simulink model "WindFoR_model"  (R2024a)
settings: Solver=VariableStepAuto  StartTime=0.0  StopTime=10.0  RelTol=1e-3
values from neighbouring files (symbols this model uses):
  b = 37.4*0.3048    (= 11.39952)    [a1_initialize.m]
  cbar = 11.52*0.3048    (= 3.511296)    [a1_initialize.m]
  g = 9.80665    [a1_initialize.m]
  InertiaTensor = [Ixx 0 -Ixz; 0 Iyy 0; -Ixz 0 Izz]    [a1_initialize.m]
  init_eulers = x0(7:9)    [a1_initialize.m]
  init_inertial = x0(10:12)    [a1_initialize.m]
  mass = 36100/2.2046    (= 16374.852581)    [a1_initialize.m]
  max_thrust = 32000*g/2.2046    (= 142344.5523)    [a1_initialize.m]
  S = 400.0*0.3048*0.3048    (= 37.161216)    [a1_initialize.m]
undefined symbols (not defined in the file or in its folder): CD0, CDalpha, CDelevator, CL0, Clalieron, CLalpha, CLalpha_dot, Clbeta, CLelevator, Clp, CLq, Clr, Clrudder, Cm0, Cmalpha, Cmalpha_dot, Cmelevator, Cmq, Cnalieron, Cnbeta, Cnp, Cnr, Cnrudder, CYalieron, CYbeta, CYp, CYr, CYrudder
libraries: Rotation_Matrices_All x2, matrix_library x2
settings Model: Creator=ragup  LastModifiedBy=ragup

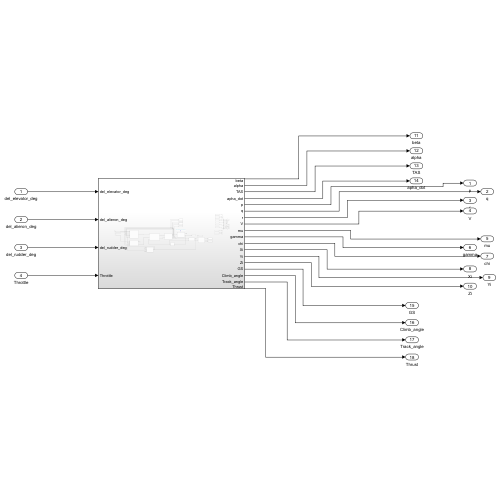
[thumbnail: Simulink's stored preview of the top-level diagram]
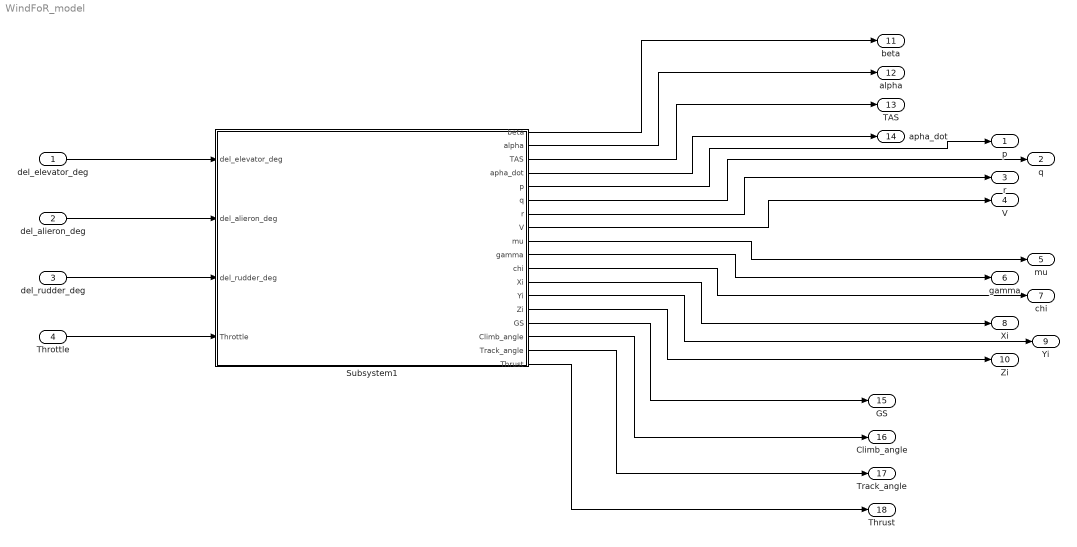
== system WindFoR_model ==
  del_elevator_deg : Inport
  del_alieron_deg : Inport  Port=2
  del_rudder_deg : Inport  Port=3
  Throttle : Inport  Port=4
  Subsystem1 : Subsystem
  p : Outport
  q : Outport  Port=2
  r : Outport  Port=3
  V : Outport  Port=4
  mu : Outport  Port=5
  gamma : Outport  Port=6
  chi : Outport  Port=7
  Xi : Outport  Port=8
  Yi : Outport  Port=9
  Zi : Outport  Port=10
  beta : Outport  Port=11
  alpha : Outport  Port=12
  TAS : Outport  Port=13
  apha_dot : Outport  Port=14
  GS : Outport  Port=15
  Climb_angle : Outport  Port=16
  Track_angle : Outport  Port=17
  Thrust : Outport  Port=18
  wires:
  del_elevator_deg/1 -> Subsystem1/1(del_elevator_deg)
  del_alieron_deg/1 -> Subsystem1/2(del_alieron_deg)
  del_rudder_deg/1 -> Subsystem1/3(del_rudder_deg)
  Throttle/1 -> Subsystem1/4(Throttle)
  Subsystem1/1(beta) -> beta/1
  Subsystem1/2(alpha) -> alpha/1
  Subsystem1/3(TAS) -> TAS/1
  Subsystem1/4(apha_dot) -> apha_dot/1
  Subsystem1/5(p) -> p/1
  Subsystem1/6(q) -> q/1
  Subsystem1/7(r) -> r/1
  Subsystem1/8(V) -> V/1
  Subsystem1/9(mu) -> mu/1
  Subsystem1/10(gamma) -> gamma/1
  Subsystem1/11(chi) -> chi/1
  Subsystem1/12(Xi) -> Xi/1
  Subsystem1/13(Yi) -> Yi/1
  Subsystem1/14(Zi) -> Zi/1
  Subsystem1/15(GS) -> GS/1
  Subsystem1/16(Climb_angle) -> Climb_angle/1
  Subsystem1/17(Track_angle) -> Track_angle/1
  Subsystem1/18(Thrust) -> Thrust/1

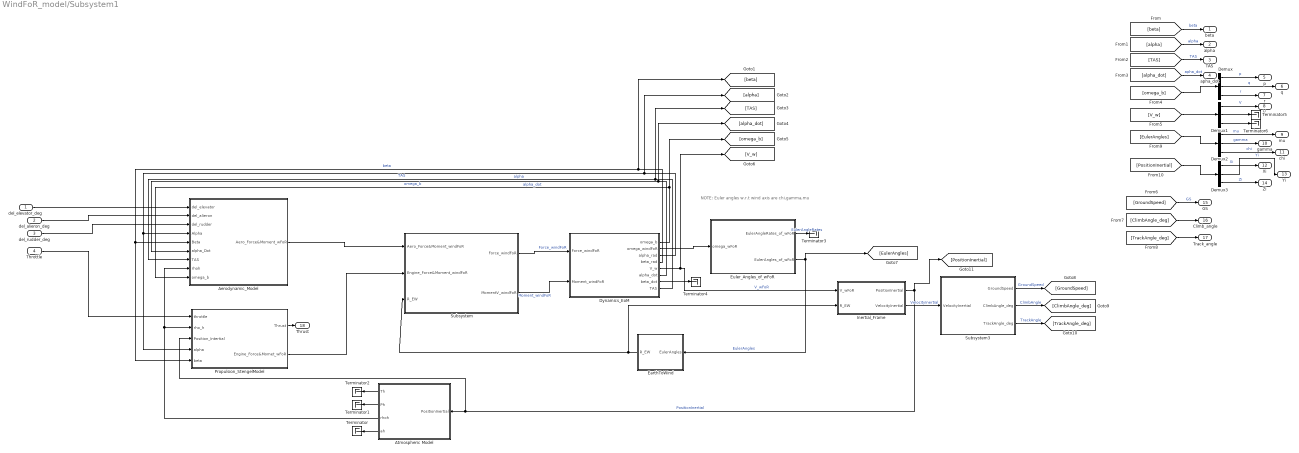
== system WindFoR_model/Subsystem1 ==
  note: NOTE: Euler angles w.r.t wind axis are chi,gamma,mu
  del_elevator_deg : Inport
  del_alieron_deg : Inport  Port=2
  del_rudder_deg : Inport  Port=3
  Throttle : Inport  Port=4
  Aerodynamic_Model : Subsystem
  Atmospheric Model : Subsystem
  Demux{,1..3} (4 alike) : Demux  Outputs=3
  Dynamics_EoM : Subsystem
  EarthToWind : Subsystem
  Euler_Angles_of_wFoR : Subsystem
  Inertial_Frame : Subsystem
  Propulsion_StengelModel : Subsystem
  Subsystem : Subsystem
  Subsystem3 : Subsystem
  Terminator{,1..6} (7 alike) : Terminator
  beta : Outport
  alpha : Outport  Port=2
  TAS : Outport  Port=3
  apha_dot : Outport  Port=4
  p : Outport  Port=5
  q : Outport  Port=6
  r : Outport  Port=7
  V : Outport  Port=8
  mu : Outport  Port=9
  gamma : Outport  Port=10
  chi : Outport  Port=11
  Xi : Outport  Port=12
  Yi : Outport  Port=13
  Zi : Outport  Port=14
  GS : Outport  Port=15
  Climb_angle : Outport  Port=16
  Track_angle : Outport  Port=17
  Thrust : Outport  Port=18
  wires:
  [alpha] -> alpha/1  "alpha"
  [EulerAngles] -> Demux2/1
  Dynamics_EoM/5(V_w) -> [V_w], Inertial_Frame/1(V_wFoR)  "V_wFoR"
  Dynamics_EoM/8(TAS) -> [TAS], Aerodynamic_Model/7(TAS)  "TAS"
  Euler_Angles_of_wFoR/2(EulerAngles_of_wFoR) -> [EulerAngles], EarthToWind/1(EulerAngles)  "EulerAngles"
  [beta] -> beta/1  "beta"
  Dynamics_EoM/4(beta_rad) -> [beta], Aerodynamic_Model/5(Beta), Propulsion_StengelModel/5(beta)  "beta"
  Propulsion_StengelModel/1(Thrust) -> Thrust/1
  Dynamics_EoM/3(alpha_rad) -> [alpha], Aerodynamic_Model/4(Alpha), Propulsion_StengelModel/4(alpha)  "alpha"
  Atmospheric Model/2(Ph) -> Terminator1/1
  Demux1/2 -> Terminator5/1
  Atmospheric Model/4(ah) -> Terminator/1
  [TrackAngle_deg] -> Track_angle/1
  [GroundSpeed] -> GS/1  "GS"
  Dynamics_EoM/7(beta_dot) -> Terminator4/1
  Subsystem3/2(ClimbAngle_deg) -> [ClimbAngle_deg]  "ClimbAngle"
  Demux/3 -> r/1  "r"
  [omega_b] -> Demux/1
  Atmospheric Model/1(Th) -> Terminator2/1
  Demux1/3 -> Terminator6/1
  [alpha_dot] -> apha_dot/1  "apha_dot"
  Demux3/2 -> Yi/1  "Yi"
  Subsystem/1(Force_windFoR) -> Dynamics_EoM/1(Force_windFoR)  "Force_windFoR"
  Demux2/2 -> gamma/1  "gamma"
  Demux1/1 -> V/1  "V"
  Demux/2 -> q/1  "q"
  [PositionInertial] -> Demux3/1
  Demux3/1 -> Xi/1  "Xi"
  del_alieron_deg/1 -> Aerodynamic_Model/2(del_alieron)
  Atmospheric Model/3(rhoh) -> Propulsion_StengelModel/2(rho_h), Aerodynamic_Model/8(rhoh)
  Euler_Angles_of_wFoR/1(EulerAngleRates_of_wFoR) -> Terminator3/1  "EulerAngleRates"
  Subsystem3/1(GroundSpeed) -> [GroundSpeed]  "GroundSpeed"
  Demux2/3 -> chi/1  "chi"
  Dynamics_EoM/1(omega_b) -> [omega_b], Aerodynamic_Model/9(omega_b)  "omega_b"
  Propulsion_StengelModel/2(Engine_Force&Momet_wFoR) -> Subsystem/2(Engine_Force&Moment_windFoR)
  Demux2/1 -> mu/1  "mu"
  Dynamics_EoM/6(alpha_dot) -> [alpha_dot], Aerodynamic_Model/6(alpha_Dot)  "alpha_dot"
  del_elevator_deg/1 -> Aerodynamic_Model/1(del_elevator)
  Inertial_Frame/2(VelocityInertial) -> Subsystem3/1(VelocityInertial)  "VelocityInertial"
  del_rudder_deg/1 -> Aerodynamic_Model/3(del_rudder)
  EarthToWind/1(R_EW) -> Inertial_Frame/2(R_EW), Subsystem/3(R_EW)
  Subsystem/2(MomentV_windFoR) -> Dynamics_EoM/2(Moment_windFoR)  "Moment_windFoR"
  Demux3/3 -> Zi/1  "Zi"
  Aerodynamic_Model/1(Aero_Force&Moment_wFoR) -> Subsystem/1(Aero_Force&Moment_windFoR)
  [TAS] -> TAS/1  "TAS"
  Subsystem3/3(TrackAngle_deg) -> [TrackAngle_deg]  "TrackAngle"
  Inertial_Frame/1(PositionInertial) -> [PositionInertial], Propulsion_StengelModel/3(Position_Intertial), Atmospheric Model/1(PositionInertial)  "PositionInertial"
  Dynamics_EoM/2(omega_windFoR) -> Euler_Angles_of_wFoR/1(omega_wFoR)
  [ClimbAngle_deg] -> Climb_angle/1
  Throttle/1 -> Propulsion_StengelModel/1(throttle)
  [V_w] -> Demux1/1
  Demux/1 -> p/1  "p"

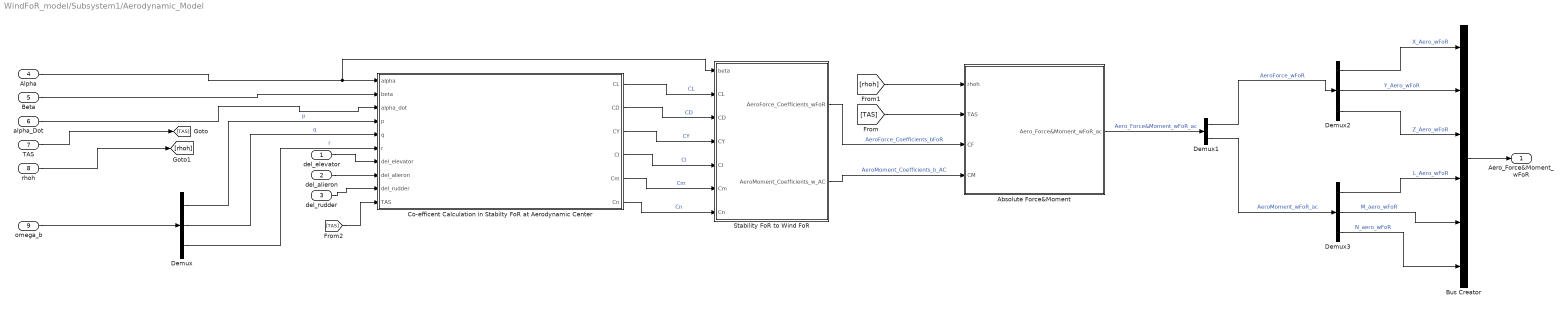
== system WindFoR_model/Subsystem1/Aerodynamic_Model ==
  del_elevator : Inport
  del_alieron : Inport  Port=2
  del_rudder : Inport  Port=3
  Alpha : Inport  Port=4
  Beta : Inport  Port=5
  alpha_Dot : Inport  Port=6
  TAS : Inport  Port=7
  rhoh : Inport  Port=8
  omega_b : Inport  Port=9
  Absolute Force&Moment : Subsystem
  Bus Creator : BusCreator  Inputs=6
  Co-efficent Calculation in Stabilty FoR at Aerodynamic Center : Subsystem
  Demux : Demux  Outputs=3
  Demux1 : Demux  Outputs=2
  Demux2 : Demux  Outputs=3
  Demux3 : Demux  Outputs=3
  Stability FoR to Wind FoR : Subsystem
  Aero_Force&Moment_wFoR : Outport
  wires:
  Demux/1 -> Co-efficent Calculation in Stabilty FoR at Aerodynamic Center/4(p)  "p"
  omega_b/1 -> Demux/1
  [TAS] -> Co-efficent Calculation in Stabilty FoR at Aerodynamic Center/10(TAS)
  TAS/1 -> [TAS]
  rhoh/1 -> [rhoh]
  Demux/2 -> Co-efficent Calculation in Stabilty FoR at Aerodynamic Center/5(q)  "q"
  Alpha/1 -> Stability FoR to Wind FoR/1(beta), Co-efficent Calculation in Stabilty FoR at Aerodynamic Center/1(alpha)
  Co-efficent Calculation in Stabilty FoR at Aerodynamic Center/1(CL) -> Stability FoR to Wind FoR/2(CL)  "CL"
  Co-efficent Calculation in Stabilty FoR at Aerodynamic Center/6(Cn) -> Stability FoR to Wind FoR/7(Cn)  "Cn"
  del_alieron/1 -> Co-efficent Calculation in Stabilty FoR at Aerodynamic Center/8(del_alieron)
  alpha_Dot/1 -> Co-efficent Calculation in Stabilty FoR at Aerodynamic Center/3(alpha_dot)
  Co-efficent Calculation in Stabilty FoR at Aerodynamic Center/3(CY) -> Stability FoR to Wind FoR/4(CY)  "CY"
  Co-efficent Calculation in Stabilty FoR at Aerodynamic Center/5(Cm) -> Stability FoR to Wind FoR/6(Cm)  "Cm"
  Co-efficent Calculation in Stabilty FoR at Aerodynamic Center/2(CD) -> Stability FoR to Wind FoR/3(CD)  "CD"
  Co-efficent Calculation in Stabilty FoR at Aerodynamic Center/4(Cl) -> Stability FoR to Wind FoR/5(Cl)  "Cl"
  Stability FoR to Wind FoR/1(AeroForce_Coefficients_wFoR) -> Absolute Force&Moment/3(CF)  "AeroForce_Coefficients_bFoR"
  [TAS] -> Absolute Force&Moment/2(TAS)
  [rhoh] -> Absolute Force&Moment/1(rhoh)
  Demux/3 -> Co-efficent Calculation in Stabilty FoR at Aerodynamic Center/6(r)  "r"
  del_elevator/1 -> Co-efficent Calculation in Stabilty FoR at Aerodynamic Center/7(del_elevator)
  Beta/1 -> Co-efficent Calculation in Stabilty FoR at Aerodynamic Center/2(beta)
  del_rudder/1 -> Co-efficent Calculation in Stabilty FoR at Aerodynamic Center/9(del_rudder)
  Stability FoR to Wind FoR/2(AeroMoment_Coefficients_w_AC) -> Absolute Force&Moment/4(CM)  "AeroMoment_Coefficients_b_AC"
  Absolute Force&Moment/1(Aero_Force&Moment_wFoR_ac) -> Demux1/1  "Aero_Force&Moment_wFoR_ac"
  Demux1/1 -> Demux2/1  "AeroForce_wFoR"
  Demux1/2 -> Demux3/1  "AeroMoment_wFoR_ac"
  Demux2/1 -> Bus Creator/1  "X_Aero_wFoR"
  Demux2/2 -> Bus Creator/2  "Y_Aero_wFoR"
  Demux2/3 -> Bus Creator/3  "Z_Aero_wFoR"
  Demux3/2 -> Bus Creator/5  "M_aero_wFoR"
  Demux3/1 -> Bus Creator/4  "L_Aero_wFoR"
  Demux3/3 -> Bus Creator/6  "N_aero_wFoR"
  Bus Creator/1 -> Aero_Force&Moment_wFoR/1

== system WindFoR_model/Subsystem1/Atmospheric Model ==
  PositionInertial : Inport
  Demux : Demux  Outputs=3
  Gain : Gain  Gain=-1
  ISA_upto20km : Subsystem
      mask Display: image('ISA_Temperature.png', [3,3,3,3,100,100]);
  Terminator : Terminator
  Terminator1 : Terminator
  Th : Outport
  Ph : Outport  Port=2
  rhoh : Outport  Port=3
  ah : Outport  Port=4
  wires:
  Demux/3 -> Gain/1
  PositionInertial/1 -> Demux/1
  ISA_upto20km/3(rhoh) -> rhoh/1  "rhoh"
  Gain/1 -> ISA_upto20km/1(h)
  Demux/2 -> Terminator1/1
  Demux/1 -> Terminator/1
  ISA_upto20km/1(Th) -> Th/1  "Th"
  ISA_upto20km/2(Ph) -> Ph/1  "Ph"
  ISA_upto20km/4(ah) -> ah/1  "ah"

== system WindFoR_model/Subsystem1/Dynamics_EoM ==
  Force_windFoR : Inport
  Moment_windFoR : Inport  Port=2
  Force_Dynamics_WindAxis : Subsystem
  Moment_Dynamics_bodyFoR : Subsystem
  Product1 : Product  Multiplication=Matrix(*)
  omega_b : Outport
  omega_windFoR : Outport  Port=2
  alpha_rad : Outport  Port=3
  beta_rad : Outport  Port=4
  V_w : Outport  Port=5
  alpha_dot : Outport  Port=6
  beta_dot : Outport  Port=7
  TAS : Outport  Port=8
  wires:
  Force_Dynamics_WindAxis/1(omega_w) -> omega_windFoR/1
  Moment_Dynamics_bodyFoR/1(omega_b) -> omega_b/1, Force_Dynamics_WindAxis/1(omega_b)  "omega_b"
  Force_Dynamics_WindAxis/8(beta_dot) -> beta_dot/1
  Force_Dynamics_WindAxis/7(alpha_dot) -> alpha_dot/1
  Force_Dynamics_WindAxis/5(V_w) -> V_w/1
  Force_Dynamics_WindAxis/4(beta_rad) -> beta_rad/1
  Force_Dynamics_WindAxis/3(alpha_rad) -> alpha_rad/1
  Product1/1 -> Moment_Dynamics_bodyFoR/1(Moment_bodyFoR)  "Moment_bodyFoR"
  Force_Dynamics_WindAxis/2(R_wb) -> [R_wb]
  Force_windFoR/1 -> Force_Dynamics_WindAxis/2(Force_w)  "Force_windFoR"
  [R_wb] -> Product1/1  "R_WB"
  Moment_windFoR/1 -> Product1/2
  Force_Dynamics_WindAxis/6(TAS) -> TAS/1

== system WindFoR_model/Subsystem1/EarthToWind ==
  EulerAngles : Inport
  Demux : Demux  Outputs=3
  Product1 : Product  Multiplication=Matrix(*)
  Product2 : Product  Multiplication=Matrix(*)
  Subsystem2 : Subsystem
  Subsystem3 : Subsystem
  Subsystem4 : Subsystem
  R_EW : Outport
  wires:
  Demux/3 -> Subsystem2/1(chi)  "chi"
  Demux/2 -> Subsystem4/1(gamma)  "gamma"
  EulerAngles/1 -> Demux/1  "EulerAngles"
  Demux/1 -> Subsystem3/1(mu)  "mu"
  Product2/1 -> R_EW/1
  Product1/1 -> Product2/1
  Subsystem2/1(R_chi) -> Product2/2
  Subsystem4/1(R_gamma) -> Product1/2
  Subsystem3/1(R_mu) -> Product1/1

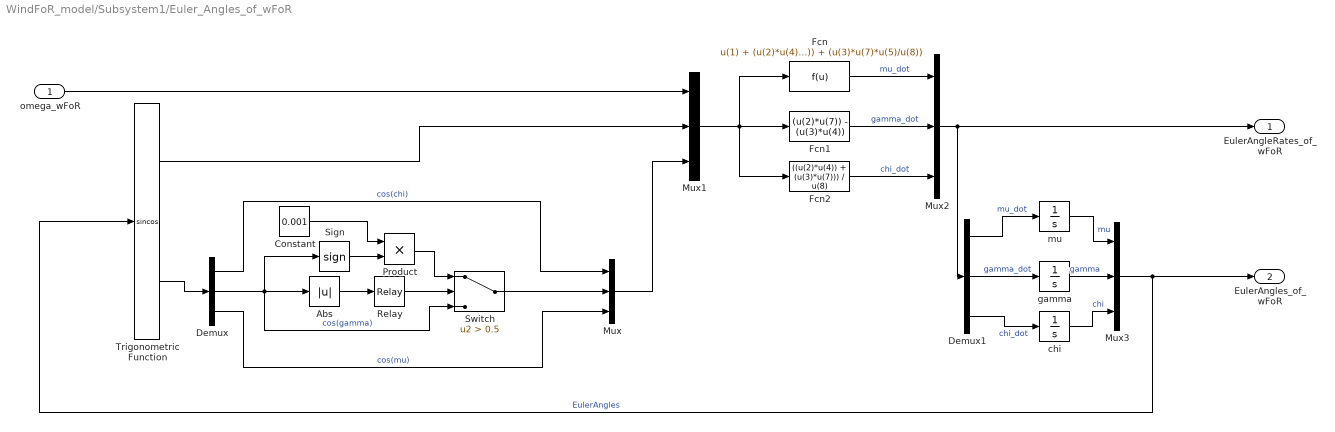
== system WindFoR_model/Subsystem1/Euler_Angles_of_wFoR ==
  omega_wFoR : Inport
  Abs : Abs  SaturateOnIntegerOverflow=off
  Constant : Constant  Value=0.001
  Demux : Demux  Outputs=3
  Demux1 : Demux  Outputs=3
  Fcn : Fcn  Expr=u(1) + (u(2)*u(4)*u(5)/u(8)) + (u(3)*u(7)*u(5)/u(8))
  Fcn1 : Fcn  Expr=(u(2)*u(7)) - (u(3)*u(4))
  Fcn2 : Fcn  Expr=((u(2)*u(4)) + (u(3)*u(7))) / u(8)
  Mux{,1..3} (4 alike) : Mux  Inputs=3
  Product : Product
  Relay : Relay  OnSwitchValue=0.001  OffSwitchValue=0  OnOutputValue=0  OffOutputValue=1
  Sign : Signum
  Switch : Switch  Criteria=u2 > Threshold  Threshold=0.5  SaturateOnIntegerOverflow=off  InputSameDT=off
  Trigonometric Function : Trigonometry  Operator=sincos
  chi : Integrator  InitialCondition=init_eulers(3)  ContinuousStateAttributes='chi'
  gamma : Integrator  InitialCondition=init_eulers(2)  ContinuousStateAttributes='gamma'
  mu : Integrator  InitialCondition=init_eulers(1)  ContinuousStateAttributes='mu'
  EulerAngleRates_of_wFoR : Outport
  EulerAngles_of_wFoR : Outport  Port=2
  wires:
  Mux3/1 -> EulerAngles_of_wFoR/1, Trigonometric Function/1  "EulerAngles"
  mu/1 -> Mux3/1  "mu"
  Demux1/3 -> chi/1  "chi_dot"
  Mux2/1 -> Demux1/1, EulerAngleRates_of_wFoR/1
  Demux1/2 -> gamma/1  "gamma_dot"
  gamma/1 -> Mux3/2  "gamma"
  Demux1/1 -> mu/1  "mu_dot"
  chi/1 -> Mux3/3  "chi"
  Fcn2/1 -> Mux2/3  "chi_dot"
  Mux/1 -> Mux1/3
  Constant/1 -> Product/1
  Demux/1 -> Mux/1  "cos(chi)"
  Fcn1/1 -> Mux2/2  "gamma_dot"
  Demux/3 -> Mux/3  "cos(mu)"
  Switch/1 -> Mux/2
  Mux1/1 -> Fcn1/1, Fcn2/1, Fcn/1
  Sign/1 -> Product/2
  Abs/1 -> Relay/1
  Fcn/1 -> Mux2/1  "mu_dot"
  Relay/1 -> Switch/2
  Product/1 -> Switch/1
  omega_wFoR/1 -> Mux1/1
  Trigonometric Function/2 -> Demux/1
  Trigonometric Function/1 -> Mux1/2
  Demux/2 -> Abs/1, Switch/3, Sign/1  "cos(gamma)"

== system WindFoR_model/Subsystem1/Inertial_Frame ==
  V_wFoR : Inport
  R_EW : Inport  Port=2
  Demux : Demux  Outputs=3
  Matrix Multiply : Product  Multiplication=Matrix(*)
  Mux : Mux  Inputs=3
  Transpose : Math  Operator=transpose
  Xi_dot : Integrator  InitialCondition=init_inertial(1)  ContinuousStateAttributes='Xi_dot'
  Yi_dot : Integrator  InitialCondition=init_inertial(2)  ContinuousStateAttributes='Yi_dot'
  Zi_dot : Integrator  InitialCondition=init_inertial(3)  ContinuousStateAttributes='Zi_dot'
  PositionInertial : Outport
  VelocityInertial : Outport  Port=2
  wires:
  R_EW/1 -> Transpose/1
  Matrix Multiply/1 -> Demux/1, VelocityInertial/1
  Transpose/1 -> Matrix Multiply/1  "R_WE"
  V_wFoR/1 -> Matrix Multiply/2
  Demux/3 -> Zi_dot/1  "Zi_dot"
  Mux/1 -> PositionInertial/1
  Zi_dot/1 -> Mux/3  "Zi"
  Xi_dot/1 -> Mux/1  "Xi"
  Demux/1 -> Xi_dot/1  "Xi_dot"
  Demux/2 -> Yi_dot/1  "Yi_dot"
  Yi_dot/1 -> Mux/2  "Yi"

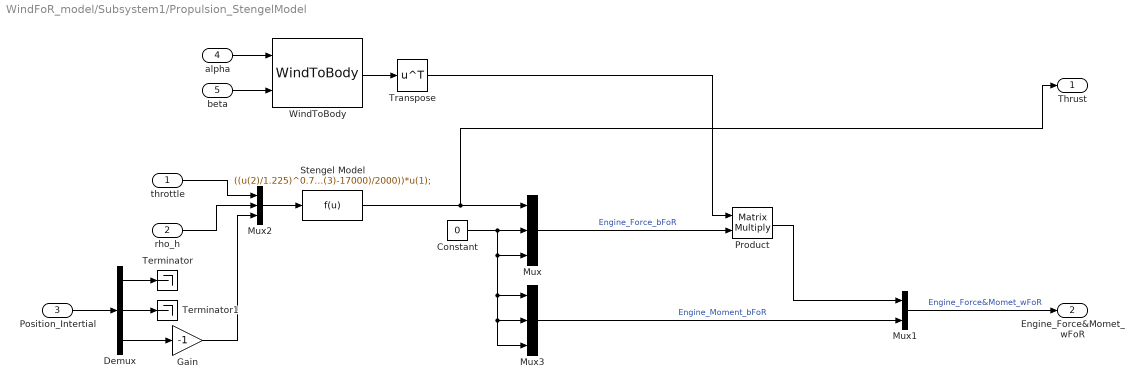
== system WindFoR_model/Subsystem1/Propulsion_StengelModel ==
  throttle : Inport
  rho_h : Inport  Port=2
  Position_Intertial : Inport  Port=3
  alpha : Inport  Port=4
  beta : Inport  Port=5
  Constant : Constant  Value=0
  Demux : Demux  Outputs=3
  Gain : Gain  Gain=-1
  Mux : Mux  Inputs=3
  Mux1 : Mux  Inputs=2
  Mux2 : Mux  Inputs=3
  Mux3 : Mux  Inputs=3
  Product : Product  Multiplication=Matrix(*)
  Stengel Model : Fcn  Expr=((u(2)/1.225)^0.7)*max_thrust*(1-exp((u(3)-17000)/2000))*u(1);
  Terminator : Terminator
  Terminator1 : Terminator
  Transpose : Math  Operator=transpose
  WindToBody : Rotation_Matrices_All/WindToBody  SystemSampleTime=-1  VariantActivationTime=update diagram  AllowFlexibleInterface=on  Latency=0  AutoFrameSizeCalculation=off
  Thrust : Outport
  Engine_Force&Momet_wFoR : Outport  Port=2
  wires:
  Stengel Model/1 -> Thrust/1, Mux/1
  Constant/1 -> Mux3/3, Mux3/2, Mux3/1, Mux/3, Mux/2
  Mux/1 -> Product/2  "Engine_Force_bFoR"
  Mux2/1 -> Stengel Model/1
  throttle/1 -> Mux2/1
  rho_h/1 -> Mux2/2
  Gain/1 -> Mux2/3
  Demux/3 -> Gain/1
  Demux/1 -> Terminator/1
  Demux/2 -> Terminator1/1
  Position_Intertial/1 -> Demux/1
  WindToBody/1 -> Transpose/1
  Transpose/1 -> Product/1
  Product/1 -> Mux1/1
  Mux1/1 -> Engine_Force&Momet_wFoR/1  "Engine_Force&Momet_wFoR"
  Mux3/1 -> Mux1/2  "Engine_Moment_bFoR"
  alpha/1 -> WindToBody/1
  beta/1 -> WindToBody/2

== system WindFoR_model/Subsystem1/Subsystem ==
  Aero_Force&Moment_windFoR : Inport
  Engine_Force&Moment_windFoR : Inport  Port=2
  R_EW : Inport  Port=3
  Add : Sum
  Constant : Constant  Value=0
  Constant1 : Constant  Value=mass
  Demux : Demux  Outputs=2
  Gain : Gain  Gain=g
  Mux : Mux  Inputs=3
  Product : Product  Multiplication=Matrix(*)
  Sum : Sum  Inputs=|++
  Force_windFoR : Outport
  MomentV_windFoR : Outport  Port=2
  wires:
  Mux/1 -> Product/2
  Demux/2 -> MomentV_windFoR/1  "Moment_windFoR"
  Add/1 -> Demux/1
  Product/1 -> Sum/1  "Gravity_Force_windFoR"
  Engine_Force&Moment_windFoR/1 -> Add/2
  Sum/1 -> Force_windFoR/1  "Force_windFoR"
  Demux/1 -> Sum/2
  Gain/1 -> Mux/3  "weight"
  Aero_Force&Moment_windFoR/1 -> Add/1
  Constant1/1 -> Gain/1
  Constant/1 -> Mux/1, Mux/2
  R_EW/1 -> Product/1

== system WindFoR_model/Subsystem1/Subsystem3 ==
  VelocityInertial : Inport
  Add : Sum
  Atan1 : Trigonometry  Operator=atan2
  Atan2 : Trigonometry  Operator=atan2
  Demux : Demux  Outputs=3
  Gain : Gain  Gain=-1
  Gain1 : Gain  Gain=180/pi
  Gain2 : Gain  Gain=180/pi
  Sqrt : Sqrt
  Square : Math  Operator=square
  Square1 : Math  Operator=square
  GroundSpeed : Outport
  ClimbAngle_deg : Outport  Port=2
  TrackAngle_deg : Outport  Port=3
  wires:
  VelocityInertial/1 -> Demux/1
  Gain/1 -> Atan2/1
  Atan1/1 -> Gain2/1
  Square/1 -> Add/1
  Demux/3 -> Gain/1  "Zdot_E"
  Add/1 -> Sqrt/1
  Atan2/1 -> Gain1/1
  Square1/1 -> Add/2
  Sqrt/1 -> Atan2/2, GroundSpeed/1
  Demux/1 -> Square/1, Atan1/2  "Xdot_E"
  Demux/2 -> Square1/1, Atan1/1  "Ydot_E"
  Gain1/1 -> ClimbAngle_deg/1
  Gain2/1 -> TrackAngle_deg/1

== system WindFoR_model/Subsystem1/Aerodynamic_Model/Absolute Force&Moment ==
  rhoh : Inport
  TAS : Inport  Port=2
  CF : Inport  Port=3
  CM : Inport  Port=4
  Constant : Constant  Value=b
  Constant1 : Constant  Value=cbar
  Demux1 : Demux  Outputs=3
  Demux2 : Demux  Outputs=3
  Mux : Mux  Inputs=6
  Product : Product
  Product1 : Product  Inputs=3
  Product2 : Product  Inputs=3
  Product3 : Product  Inputs=3
  Subsystem1 : Subsystem
  Aero_Force&Moment_wFoR_ac : Outport
  wires:
  Demux2/3 -> Product3/2
  Demux1/3 -> Mux/3  "Z_aero"
  Constant1/1 -> Product2/3
  CF/1 -> Product/2
  CM/1 -> Demux2/1
  Demux1/1 -> Mux/1  "X_aero"
  Product3/1 -> Mux/6  "N_aero"
  Subsystem1/1(QS) -> [QS]  "QS"
  Constant/1 -> Product3/3, Product1/3
  Product/1 -> Demux1/1  "Aero_Forces"
  Demux2/1 -> Product1/2  "Cl"
  Demux2/2 -> Product2/2
  [QS] -> Product3/1, Product2/1, Product1/1
  Product2/1 -> Mux/5  "M_aero"
  Demux1/2 -> Mux/2  "Y_aero"
  Product1/1 -> Mux/4  "L_aero"
  rhoh/1 -> Subsystem1/1(rhoh)
  [QS] -> Product/1
  TAS/1 -> Subsystem1/2(TAS)
  Mux/1 -> Aero_Force&Moment_wFoR_ac/1  "Aero_Force&Moment_wFoR_ac"

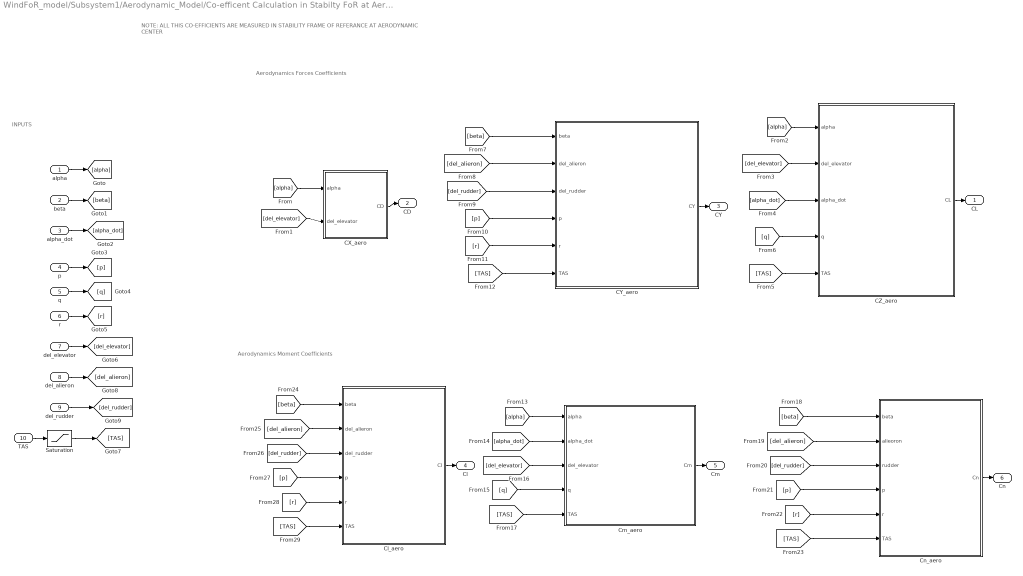
== system WindFoR_model/Subsystem1/Aerodynamic_Model/Co-efficent Calculation in Stabilty FoR at Aerodynamic Center ==
  note: INPUTS
  note: Aerodynamics Moment Coefficients
  note: Aerodynamics Forces Coefficients
  note: NOTE: ALL THIS CO-EFFICIENTS ARE MEASURED IN STABILITY FRAME OF REFERANCE AT AERODYNAMIC CENTER
  alpha : Inport
  beta : Inport  Port=2
  alpha_dot : Inport  Port=3
  p : Inport  Port=4
  q : Inport  Port=5
  r : Inport  Port=6
  del_elevator : Inport  Port=7
  del_alieron : Inport  Port=8
  del_rudder : Inport  Port=9
  TAS : Inport  Port=10
  CX_aero : Subsystem
  CY_aero : Subsystem
  CZ_aero : Subsystem
  Cl_aero : Subsystem
  Cm_aero : Subsystem
  Cn_aero : Subsystem
  Saturation : Saturate  UpperLimit=inf  LowerLimit=0.1
  CL : Outport
  CD : Outport  Port=2
  CY : Outport  Port=3
  Cl : Outport  Port=4
  Cm : Outport  Port=5
  Cn : Outport  Port=6
  wires:
  Saturation/1 -> [TAS]
  [del_elevator] -> CZ_aero/2(del_elevator)
  alpha/1 -> [alpha]
  TAS/1 -> Saturation/1
  [r] -> Cn_aero/5(r)
  [alpha] -> Cm_aero/1(alpha)
  q/1 -> [q]
  beta/1 -> [beta]
  [r] -> Cl_aero/5(r)
  del_alieron/1 -> [del_alieron]
  p/1 -> [p]
  alpha_dot/1 -> [alpha_dot]
  [q] -> Cm_aero/4(q)
  [alpha_dot] -> Cm_aero/2(alpha_dot)
  [r] -> CY_aero/5(r)
  del_rudder/1 -> [del_rudder]
  [TAS] -> CY_aero/6(TAS)
  del_elevator/1 -> [del_elevator]
  [alpha] -> CX_aero/1(alpha)
  [del_elevator] -> CX_aero/2(del_elevator)
  [del_elevator] -> Cm_aero/3(del_elevator)
  Cm_aero/1(Cm) -> Cm/1
  [del_rudder] -> Cl_aero/3(del_rudder)
  [TAS] -> Cm_aero/5(TAS)
  [TAS] -> Cl_aero/6(TAS)
  [beta] -> Cl_aero/1(beta)
  [del_rudder] -> Cn_aero/3(rudder)
  [beta] -> CY_aero/1(beta)
  [p] -> Cl_aero/4(p)
  [beta] -> Cn_aero/1(beta)
  [del_alieron] -> Cl_aero/2(del_alieron)
  r/1 -> [r]
  [TAS] -> CZ_aero/5(TAS)
  Cl_aero/1(Cl) -> Cl/1
  [del_alieron] -> Cn_aero/2(alieoron)
  [p] -> Cn_aero/4(p)
  [TAS] -> Cn_aero/6(TAS)
  [alpha] -> CZ_aero/1(alpha)
  [q] -> CZ_aero/4(q)
  Cn_aero/1(Cn) -> Cn/1
  [alpha_dot] -> CZ_aero/3(alpha_dot)
  [del_alieron] -> CY_aero/2(del_alieron)
  [del_rudder] -> CY_aero/3(del_rudder)
  CX_aero/1(CD) -> CD/1
  [p] -> CY_aero/4(p)
  CY_aero/1(CY) -> CY/1
  CZ_aero/1(CL) -> CL/1

== system WindFoR_model/Subsystem1/Aerodynamic_Model/Stability FoR to Wind FoR ==
  note: Cx = -CD
      | Cz = -CL
  note: In stability FoR
      | at AC
  note: In body FoR
      | at AC
  beta : Inport
  CL : Inport  Port=2
  CD : Inport  Port=3
  CY : Inport  Port=4
  Cl : Inport  Port=5
  Cm : Inport  Port=6
  Cn : Inport  Port=7
  Demux : Demux  Outputs=3
  Gain : Gain  Gain=-1
  Gain1 : Gain  Gain=-1
  Matrix Multiply : Product  Multiplication=Matrix(*)
  Matrix Multiply1 : Product  Multiplication=Matrix(*)
  Mux : Mux  Inputs=3
  Mux1 : Mux  Inputs=3
  Mux2 : Mux  Inputs=3
  StabilityToWind : Rotation_Matrices_All/StabilityToWind  SystemSampleTime=-1  VariantActivationTime=update diagram  AllowFlexibleInterface=on  Latency=0  AutoFrameSizeCalculation=off
  AeroForce_Coefficients_wFoR : Outport
  AeroMoment_Coefficients_w_AC : Outport  Port=2
  wires:
  Mux/1 -> Matrix Multiply/2  "AeroForce_Coefficients_sFoR"
  Cm/1 -> Mux1/2
  StabilityToWind/1 -> Matrix Multiply1/1, Matrix Multiply/1
  Mux1/1 -> Matrix Multiply1/2  "AeroMoment_Coefficients_sFoR"
  beta/1 -> StabilityToWind/1
  Cn/1 -> Mux1/3
  Cl/1 -> Mux1/1
  Matrix Multiply1/1 -> AeroMoment_Coefficients_w_AC/1  "AeroMoment_Coefficients_w_AC"
  CD/1 -> Mux/1
  CY/1 -> Mux/2
  CL/1 -> Mux/3
  Matrix Multiply/1 -> Demux/1
  Demux/1 -> Gain/1
  Mux2/1 -> AeroForce_Coefficients_wFoR/1  "AeroForce_Coefficients_wFoR"
  Gain/1 -> Mux2/1
  Demux/2 -> Mux2/2
  Demux/3 -> Gain1/1
  Gain1/1 -> Mux2/3

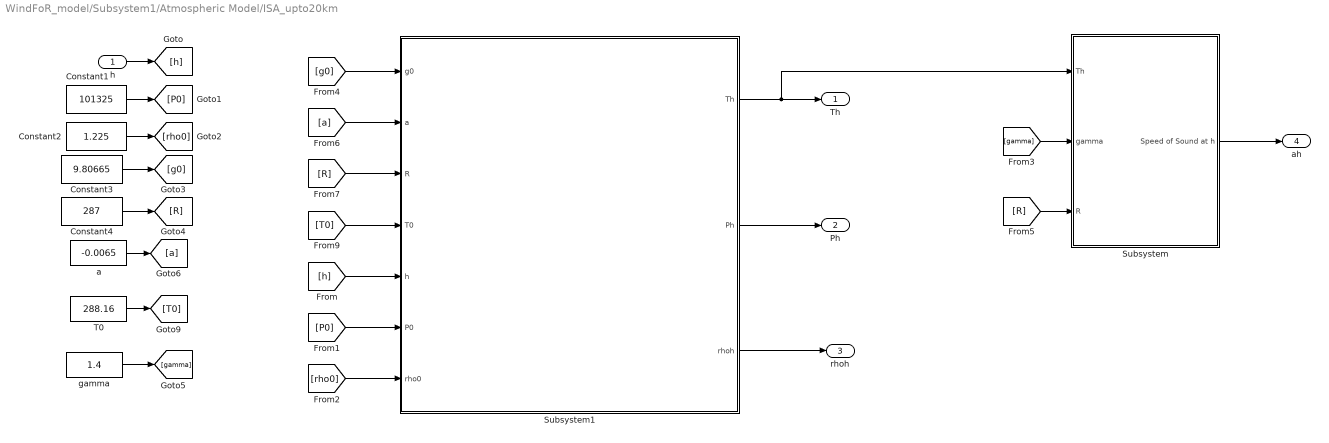
== system WindFoR_model/Subsystem1/Atmospheric Model/ISA_upto20km ==
  h : Inport
  Constant1 : Constant  Value=101325
  Constant2 : Constant  Value=1.225
  Constant3 : Constant  Value=9.80665
  Constant4 : Constant  Value=287
  Subsystem : Subsystem
  Subsystem1 : Subsystem
  T0 : Constant  Value=288.16
  a : Constant  Value=-0.0065
  gamma : Constant  Value=1.4
  Th : Outport
  Ph : Outport  Port=2
  rhoh : Outport  Port=3
  ah : Outport  Port=4
  wires:
  gamma/1 -> [gamma]
  a/1 -> [a]
  Constant1/1 -> [P0]
  Constant4/1 -> [R]
  Constant2/1 -> [rho0]
  Constant3/1 -> [g0]
  h/1 -> [h]
  T0/1 -> [T0]
  [g0] -> Subsystem1/1(g0)
  [a] -> Subsystem1/2(a)
  [R] -> Subsystem1/3(R)
  [T0] -> Subsystem1/4(T0)
  [h] -> Subsystem1/5(h)
  [P0] -> Subsystem1/6(P0)
  [rho0] -> Subsystem1/7(rho0)
  Subsystem1/1(Th) -> Subsystem/1(Th), Th/1
  Subsystem1/2(Ph) -> Ph/1
  Subsystem1/3(rhoh) -> rhoh/1
  Subsystem/1(Speed of Sound at h) -> ah/1
  [gamma] -> Subsystem/2(gamma)
  [R] -> Subsystem/3(R)

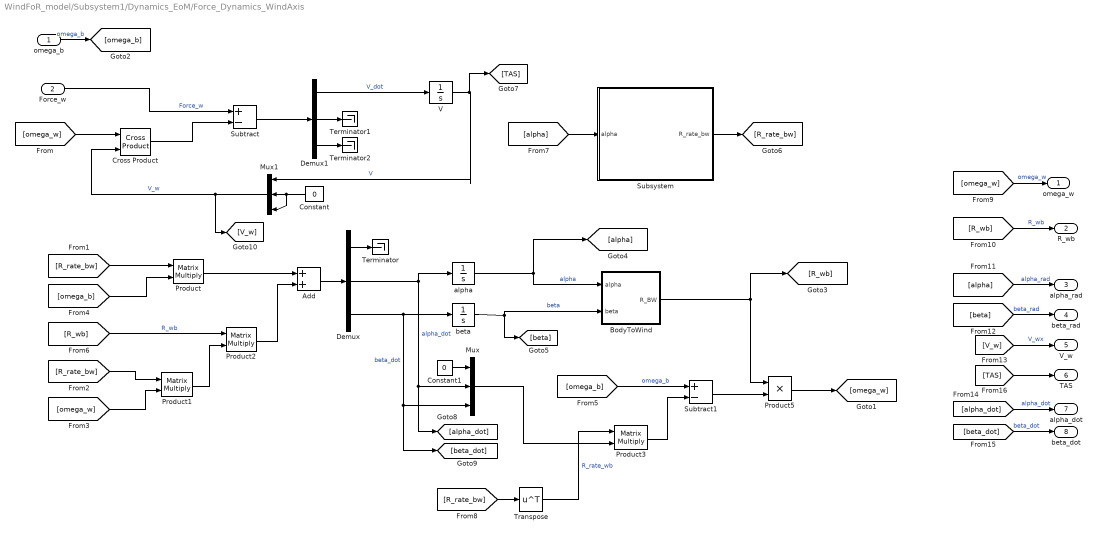
== system WindFoR_model/Subsystem1/Dynamics_EoM/Force_Dynamics_WindAxis ==
  omega_b : Inport
  Force_w : Inport  Port=2
  Add : Sum
  BodyToWind : Subsystem
  Constant : Constant  Value=0
  Constant1 : Constant  Value=0
  Cross Product : matrix_library/Cross Product
  Demux : Demux  Outputs=3
  Demux1 : Demux  Outputs=3
  Mux : Mux  Inputs=3
  Mux1 : Mux  Inputs=3
  Product{,1..3} (4 alike) : Product  Multiplication=Matrix(*)
  Product5 : Product
  Subsystem : Subsystem
  Subtract : Sum  Inputs=+-
  Subtract1 : Sum  Inputs=+-
  Terminator : Terminator
  Terminator1 : Terminator
  Terminator2 : Terminator
  Transpose : Math  Operator=transpose
  V : Integrator
  alpha : Integrator
  beta : Integrator
  omega_w : Outport
  R_wb : Outport  Port=2
  alpha_rad : Outport  Port=3
  beta_rad : Outport  Port=4
  V_w : Outport  Port=5
  TAS : Outport  Port=6
  alpha_dot : Outport  Port=7
  beta_dot : Outport  Port=8
  wires:
  Subsystem/1(R_rate_bw) -> [R_rate_bw]
  alpha/1 -> BodyToWind/1(alpha), [alpha]  "alpha"
  Transpose/1 -> Product3/1  "R_rate_wb"
  Demux1/2 -> Terminator1/1
  Product5/1 -> [omega_w]
  V/1 -> [TAS], Mux1/1  "V"
  [omega_w] -> Product1/2
  [R_rate_bw] -> Product1/1
  Demux/1 -> Terminator/1
  [alpha] -> Subsystem/1(alpha)
  Product/1 -> Add/1
  Product1/1 -> Product2/2
  Demux/3 -> [beta_dot], Mux/3, beta/1  "beta_dot"
  Product2/1 -> Add/2
  Demux1/3 -> Terminator2/1
  [R_rate_bw] -> Product/1
  Demux/2 -> [alpha_dot], Mux/2, alpha/1  "alpha_dot"
  Product3/1 -> Subtract1/2
  beta/1 -> [beta], BodyToWind/2(beta)  "beta"
  Force_w/1 -> Subtract/1  "Force_w"
  Constant1/1 -> Mux/1
  Constant/1 -> Mux1/3, Mux1/2
  [omega_w] -> Cross Product/1
  Cross Product/1 -> Subtract/2
  [omega_b] -> Product/2
  omega_b/1 -> [omega_b]  "omega_b"
  Mux/1 -> Product3/2
  [R_wb] -> Product2/1  "R_wb"
  Subtract/1 -> Demux1/1
  [omega_b] -> Subtract1/1  "omega_b"
  BodyToWind/1(R_BW) -> Product5/1, [R_wb]
  Mux1/1 -> [V_w], Cross Product/2  "V_w"
  Demux1/1 -> V/1  "V_dot"
  Add/1 -> Demux/1
  [R_rate_bw] -> Transpose/1
  Subtract1/1 -> Product5/2
  [omega_w] -> omega_w/1  "omega_w"
  [R_wb] -> R_wb/1  "R_wb"
  [alpha] -> alpha_rad/1  "alpha_rad"
  [beta] -> beta_rad/1  "beta_rad"
  [V_w] -> V_w/1  "V_wx"
  [alpha_dot] -> alpha_dot/1  "alpha_dot"
  [beta_dot] -> beta_dot/1  "beta_dot"
  [TAS] -> TAS/1

== system WindFoR_model/Subsystem1/Dynamics_EoM/Moment_Dynamics_bodyFoR ==
  Moment_bodyFoR : Inport
  Add : Sum  Inputs=+-
  Constant : Constant  Value=InertiaTensor
  Cross Product : matrix_library/Cross Product
  Demux : Demux  Outputs=3
  Divide : Product  Inputs=/*  Multiplication=Matrix(*)
  Mux : Mux  Inputs=3
  Product : Product  Multiplication=Matrix(*)
  p_dot : Integrator  ContinuousStateAttributes='p_dot'
  q_dot : Integrator  ContinuousStateAttributes='q_dot'
  r_dot : Integrator  ContinuousStateAttributes='r_dot'
  omega_b : Outport
  wires:
  Divide/1 -> Demux/1
  r_dot/1 -> Mux/3  "r"
  p_dot/1 -> Mux/1  "p"
  Product/1 -> Cross Product/2
  Demux/2 -> q_dot/1  "q_dot"
  Mux/1 -> omega_b/1, Product/2, Cross Product/1  "omega_b"
  Add/1 -> Divide/2
  Cross Product/1 -> Add/2
  Demux/3 -> r_dot/1  "r_dot"
  q_dot/1 -> Mux/2  "q"
  Demux/1 -> p_dot/1  "p_dot"
  Constant/1 -> Divide/1, Product/1
  Moment_bodyFoR/1 -> Add/1

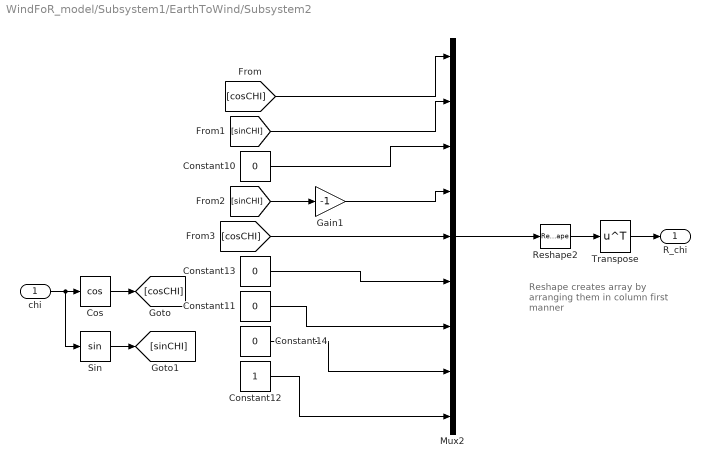
== system WindFoR_model/Subsystem1/EarthToWind/Subsystem2 ==
  note: Reshape creates array by arranging them in column first manner
  chi : Inport
  Constant{10..11,13..14} (4 alike) : Constant  Value=0
  Constant12 : Constant
  Cos : Trigonometry  Operator=cos
  Gain1 : Gain  Gain=-1
  Mux2 : Mux  Inputs=9
  Reshape2 : Reshape  OutputDimensionality=Customize  OutputDimensions=[3,3]
  Sin : Trigonometry
  Transpose : Math  Operator=transpose
  R_chi : Outport
  wires:
  Transpose/1 -> R_chi/1
  [cosCHI] -> Mux2/5
  Gain1/1 -> Mux2/4
  Constant11/1 -> Mux2/7
  Constant14/1 -> Mux2/8
  Constant12/1 -> Mux2/9
  Constant13/1 -> Mux2/6
  Mux2/1 -> Reshape2/1
  Reshape2/1 -> Transpose/1
  Sin/1 -> [sinCHI]
  Cos/1 -> [cosCHI]
  Constant10/1 -> Mux2/3
  [cosCHI] -> Mux2/1
  [sinCHI] -> Gain1/1
  [sinCHI] -> Mux2/2
  chi/1 -> Cos/1, Sin/1

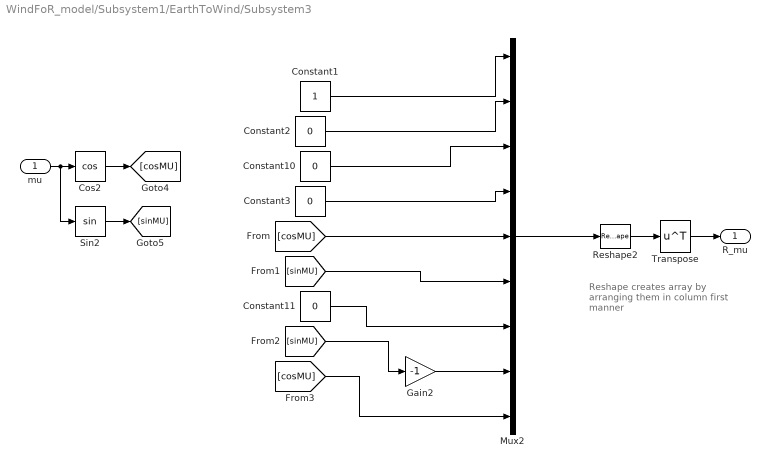
== system WindFoR_model/Subsystem1/EarthToWind/Subsystem3 ==
  note: Reshape creates array by arranging them in column first manner
  mu : Inport
  Constant1 : Constant
  Constant{2..3,10..11} (4 alike) : Constant  Value=0
  Cos2 : Trigonometry  Operator=cos
  Gain2 : Gain  Gain=-1
  Mux2 : Mux  Inputs=9
  Reshape2 : Reshape  OutputDimensionality=Customize  OutputDimensions=[3,3]
  Sin2 : Trigonometry
  Transpose : Math  Operator=transpose
  R_mu : Outport
  wires:
  Gain2/1 -> Mux2/8
  Cos2/1 -> [cosMU]
  Sin2/1 -> [sinMU]
  mu/1 -> Cos2/1, Sin2/1
  Constant2/1 -> Mux2/2
  Constant1/1 -> Mux2/1
  Constant10/1 -> Mux2/3
  Reshape2/1 -> Transpose/1
  Mux2/1 -> Reshape2/1
  [sinMU] -> Mux2/6
  [cosMU] -> Mux2/9
  [sinMU] -> Gain2/1
  Constant11/1 -> Mux2/7
  Constant3/1 -> Mux2/4
  [cosMU] -> Mux2/5
  Transpose/1 -> R_mu/1

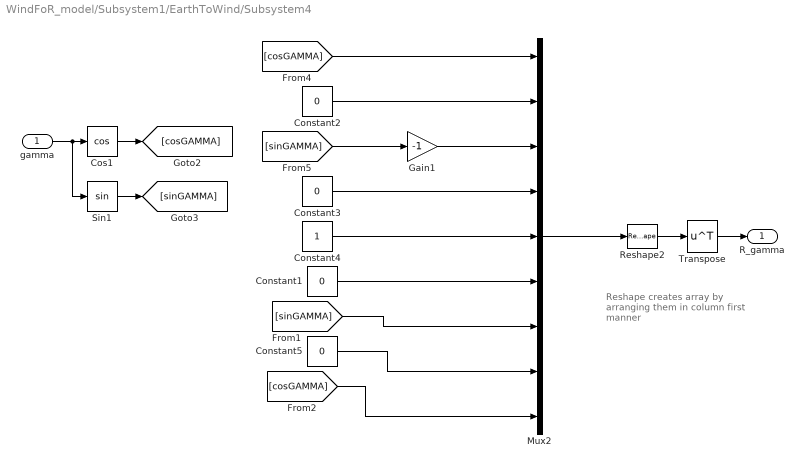
== system WindFoR_model/Subsystem1/EarthToWind/Subsystem4 ==
  note: Reshape creates array by arranging them in column first manner
  gamma : Inport
  Constant{1..3,5} (4 alike) : Constant  Value=0
  Constant4 : Constant
  Cos1 : Trigonometry  Operator=cos
  Gain1 : Gain  Gain=-1
  Mux2 : Mux  Inputs=9
  Reshape2 : Reshape  OutputDimensionality=Customize  OutputDimensions=[3,3]
  Sin1 : Trigonometry
  Transpose : Math  Operator=transpose
  R_gamma : Outport
  wires:
  Gain1/1 -> Mux2/3
  Cos1/1 -> [cosGAMMA]
  gamma/1 -> Cos1/1, Sin1/1
  Sin1/1 -> [sinGAMMA]
  Transpose/1 -> R_gamma/1
  Constant4/1 -> Mux2/5
  Constant3/1 -> Mux2/4
  [sinGAMMA] -> Mux2/7
  [cosGAMMA] -> Mux2/9
  Constant1/1 -> Mux2/6
  Mux2/1 -> Reshape2/1
  Reshape2/1 -> Transpose/1
  [sinGAMMA] -> Gain1/1
  [cosGAMMA] -> Mux2/1
  Constant2/1 -> Mux2/2
  Constant5/1 -> Mux2/8

== system WindFoR_model/Subsystem1/Aerodynamic_Model/Absolute Force&Moment/Subsystem1 ==
  rhoh : Inport
  TAS : Inport  Port=2
  Gain : Gain  Gain=1/2
  Product : Product
  Product1 : Product
  Square : Math  Operator=square
  WingArea : Constant  Value=S
  QS : Outport
  wires:
  TAS/1 -> Square/1
  Product/1 -> Product1/2  "Q"
  rhoh/1 -> Gain/1
  Gain/1 -> Product/1
  WingArea/1 -> Product1/1
  Product1/1 -> QS/1  "QS"
  Square/1 -> Product/2

== system WindFoR_model/Subsystem1/Aerodynamic_Model/Co-efficent Calculation in Stabilty FoR at Aerodynamic Center/CX_aero ==
  alpha : Inport
  del_elevator : Inport  Port=2
  Abs : Abs  SaturateOnIntegerOverflow=off
  Abs1 : Abs  SaturateOnIntegerOverflow=off
  Add : Sum  Inputs=+++
  CDalpha : Gain  Gain=CDalpha
  CDelevator : Gain  Gain=CDelevator
  Constant : Constant  Value=CD0
  CD : Outport
  wires:
  CDalpha/1 -> Add/2
  Constant/1 -> Add/1
  CDelevator/1 -> Add/3
  Add/1 -> CD/1  "CD"
  alpha/1 -> Abs/1
  del_elevator/1 -> Abs1/1
  Abs/1 -> CDalpha/1
  Abs1/1 -> CDelevator/1

== system WindFoR_model/Subsystem1/Aerodynamic_Model/Co-efficent Calculation in Stabilty FoR at Aerodynamic Center/CY_aero ==
  beta : Inport
  del_alieron : Inport  Port=2
  del_rudder : Inport  Port=3
  p : Inport  Port=4
  r : Inport  Port=5
  TAS : Inport  Port=6
  Add : Sum  Inputs=+++++
  CYalieron : Gain  Gain=CYalieron
  CYbeta : Gain  Gain=CYbeta
  CYp : Gain  Gain=CYp
  CYr : Gain  Gain=CYr
  CYrudder : Gain  Gain=CYrudder
  Constant1 : Constant  Value=b/2
  Divide : Product  Inputs=*/
  Product : Product
  Product1 : Product
  CY : Outport
  wires:
  CYalieron/1 -> Add/2
  Divide/1 -> Product1/2, Product/2
  Product1/1 -> Add/5
  del_rudder/1 -> CYrudder/1
  CYr/1 -> Product1/1
  Constant1/1 -> Divide/1
  p/1 -> CYp/1
  del_alieron/1 -> CYalieron/1
  CYbeta/1 -> Add/1
  CYrudder/1 -> Add/3
  CYp/1 -> Product/1
  Product/1 -> Add/4
  Add/1 -> CY/1  "CY"
  TAS/1 -> Divide/2
  r/1 -> CYr/1
  beta/1 -> CYbeta/1

== system WindFoR_model/Subsystem1/Aerodynamic_Model/Co-efficent Calculation in Stabilty FoR at Aerodynamic Center/CZ_aero ==
  alpha : Inport
  del_elevator : Inport  Port=2
  alpha_dot : Inport  Port=3
  q : Inport  Port=4
  TAS : Inport  Port=5
  Add : Sum  Inputs=+++++
  AvioidDivByZero : Saturate  UpperLimit=inf  LowerLimit=0.1
  CLalpha : Gain  Gain=CLalpha
  CLalpha_dot : Gain  Gain=CLalpha_dot
  CLelevator : Gain  Gain=CLelevator
  CLq : Gain  Gain=CLq
  Constant : Constant  Value=CL0
  Constant1 : Constant  Value=cbar/2
  Divide : Product  Inputs=*/
  Product : Product
  Product1 : Product
  CL : Outport
  wires:
  AvioidDivByZero/1 -> Divide/2
  CLalpha/1 -> Add/2
  CLelevator/1 -> Add/3
  Product1/1 -> Add/5
  CLq/1 -> Product1/1
  alpha/1 -> CLalpha/1
  CLalpha_dot/1 -> Product/1
  q/1 -> CLq/1
  Product/1 -> Add/4
  Add/1 -> CL/1  "CL"
  del_elevator/1 -> CLelevator/1
  Constant/1 -> Add/1
  alpha_dot/1 -> CLalpha_dot/1
  TAS/1 -> AvioidDivByZero/1
  Constant1/1 -> Divide/1
  Divide/1 -> Product1/2, Product/2

== system WindFoR_model/Subsystem1/Aerodynamic_Model/Co-efficent Calculation in Stabilty FoR at Aerodynamic Center/Cl_aero ==
  beta : Inport
  del_alieron : Inport  Port=2
  del_rudder : Inport  Port=3
  p : Inport  Port=4
  r : Inport  Port=5
  TAS : Inport  Port=6
  Add : Sum  Inputs=+++++
  Clalieron : Gain  Gain=Clalieron
  Clbeta : Gain  Gain=Clbeta
  Clp : Gain  Gain=Clp
  Clr : Gain  Gain=Clr
  Clrudder : Gain  Gain=Clrudder
  Constant : Constant  Value=b/2
  Divide : Product  Inputs=*/
  Product : Product
  Product1 : Product
  Cl : Outport
  wires:
  Clalieron/1 -> Add/2
  Product/1 -> Add/4
  Divide/1 -> Product1/2, Product/2
  Constant/1 -> Divide/1
  p/1 -> Clp/1
  Clrudder/1 -> Add/3
  Clr/1 -> Product1/1
  Clbeta/1 -> Add/1
  Product1/1 -> Add/5
  Clp/1 -> Product/1
  TAS/1 -> Divide/2
  beta/1 -> Clbeta/1
  r/1 -> Clr/1
  del_rudder/1 -> Clrudder/1
  del_alieron/1 -> Clalieron/1
  Add/1 -> Cl/1  "Cl"

== system WindFoR_model/Subsystem1/Aerodynamic_Model/Co-efficent Calculation in Stabilty FoR at Aerodynamic Center/Cm_aero ==
  alpha : Inport
  alpha_dot : Inport  Port=2
  del_elevator : Inport  Port=3
  q : Inport  Port=4
  TAS : Inport  Port=5
  Add : Sum  Inputs=+++++
  Cm0 : Constant  Value=Cm0
  Cmalpha : Gain  Gain=Cmalpha
  Cmalpha_dot : Gain  Gain=Cmalpha_dot
  Cmelevator : Gain  Gain=Cmelevator
  Cmq : Gain  Gain=Cmq
  Constant1 : Constant  Value=cbar/2
  Divide : Product  Inputs=*/
  Product : Product
  Product1 : Product
  Cm : Outport
  wires:
  Cm0/1 -> Add/1
  Cmelevator/1 -> Add/4
  Cmq/1 -> Product/1
  Divide/1 -> Product1/2, Product/2
  alpha/1 -> Cmalpha/1
  Constant1/1 -> Divide/1
  Cmalpha/1 -> Add/2
  Product/1 -> Add/5
  TAS/1 -> Divide/2
  Add/1 -> Cm/1  "Cm"
  q/1 -> Cmq/1
  del_elevator/1 -> Cmelevator/1
  alpha_dot/1 -> Cmalpha_dot/1
  Cmalpha_dot/1 -> Product1/1
  Product1/1 -> Add/3

== system WindFoR_model/Subsystem1/Aerodynamic_Model/Co-efficent Calculation in Stabilty FoR at Aerodynamic Center/Cn_aero ==
  beta : Inport
  alieoron : Inport  Port=2
  rudder : Inport  Port=3
  p : Inport  Port=4
  r : Inport  Port=5
  TAS : Inport  Port=6
  Add : Sum  Inputs=+++++
  Cnalieron : Gain  Gain=Cnalieron
  Cnbeta : Gain  Gain=Cnbeta
  Cnp : Gain  Gain=Cnp
  Cnr : Gain  Gain=Cnr
  Cnrudder : Gain  Gain=Cnrudder
  Constant : Constant  Value=b/2
  Divide : Product  Inputs=*/
  Product : Product
  Product1 : Product
  Cn : Outport
  wires:
  Cnalieron/1 -> Add/2
  Product/1 -> Add/4
  Divide/1 -> Product1/2, Product/2
  Constant/1 -> Divide/1
  p/1 -> Cnp/1
  Cnrudder/1 -> Add/3
  Cnr/1 -> Product1/1
  Cnbeta/1 -> Add/1
  Product1/1 -> Add/5
  Cnp/1 -> Product/1
  TAS/1 -> Divide/2
  beta/1 -> Cnbeta/1
  r/1 -> Cnr/1
  rudder/1 -> Cnrudder/1
  alieoron/1 -> Cnalieron/1
  Add/1 -> Cn/1  "Cn"

== system WindFoR_model/Subsystem1/Atmospheric Model/ISA_upto20km/Subsystem ==
  Th : Inport
  gamma : Inport  Port=2
  R : Inport  Port=3
  Product : Product
  Product1 : Product
  Sqrt : Sqrt
  Speed of Sound at h : Outport
  wires:
  R/1 -> Product/2
  Th/1 -> Product1/1
  Product1/1 -> Sqrt/1
  Sqrt/1 -> Speed of Sound at h/1
  Product/1 -> Product1/2
  gamma/1 -> Product/1

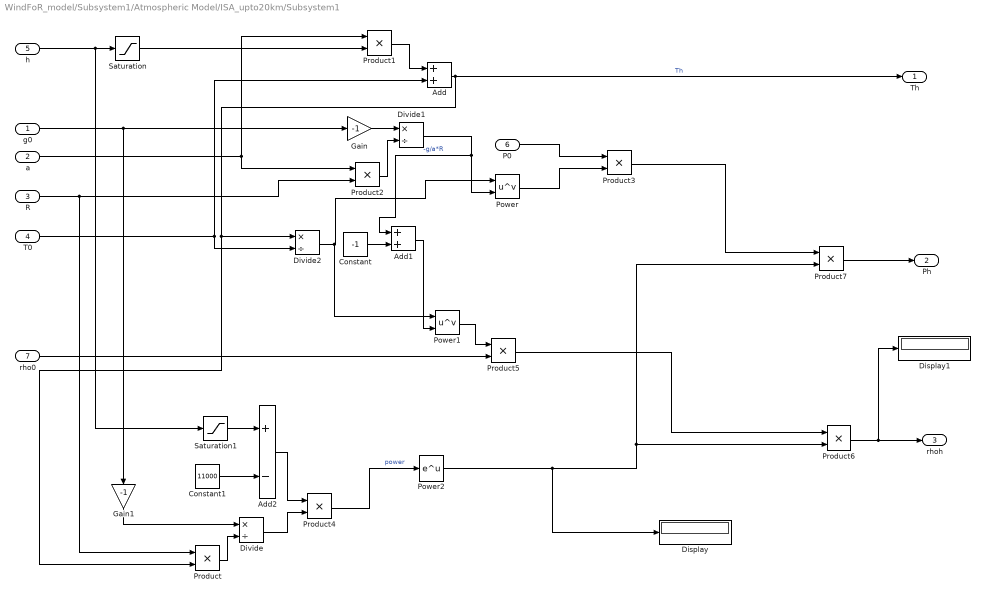
== system WindFoR_model/Subsystem1/Atmospheric Model/ISA_upto20km/Subsystem1 ==
  g0 : Inport
  a : Inport  Port=2
  R : Inport  Port=3
  T0 : Inport  Port=4
  h : Inport  Port=5
  P0 : Inport  Port=6
  rho0 : Inport  Port=7
  Add : Sum
  Add1 : Sum
  Add2 : Sum  Inputs=+-
  Constant : Constant  Value=-1
  Constant1 : Constant  Value=11000
  Display : Display
  Display1 : Display
  Divide : Product  Inputs=*/
  Divide1 : Product  Inputs=*/
  Divide2 : Product  Inputs=*/
  Gain : Gain  Gain=-1
  Gain1 : Gain  Gain=-1
  Power : Math  Operator=pow
  Power1 : Math  Operator=pow
  Power2 : Math
  Product{,1..7} (8 alike) : Product
  Saturation : Saturate  UpperLimit=11000  LowerLimit=0
  Saturation1 : Saturate  UpperLimit=25000  LowerLimit=11000
  Th : Outport
  Ph : Outport  Port=2
  rhoh : Outport  Port=3
  wires:
  Divide2/1 -> Power1/1, Power/1
  Divide1/1 -> Power/2, Add1/1  "-g/a*R"
  Product3/1 -> Product7/1
  Power/1 -> Product3/2
  Product2/1 -> Divide1/2
  Constant/1 -> Add1/2
  Gain/1 -> Divide1/1
  R/1 -> Product/1, Product2/2
  Power1/1 -> Product5/1
  rho0/1 -> Product5/2
  P0/1 -> Product3/1
  Add1/1 -> Power1/2
  g0/1 -> Gain1/1, Gain/1
  a/1 -> Product2/1, Product1/1
  Product5/1 -> Product6/1
  h/1 -> Saturation1/1, Saturation/1
  Product1/1 -> Add/1
  Add/1 -> Th/1, Product/2, Divide2/1  "Th"
  Saturation/1 -> Product1/2
  Saturation1/1 -> Add2/1
  Add2/1 -> Product4/1
  Constant1/1 -> Add2/2
  Product/1 -> Divide/2
  Divide/1 -> Product4/2
  Product4/1 -> Power2/1  "power"
  Power2/1 -> Display/1, Product6/2, Product7/2
  T0/1 -> Divide2/2, Add/2
  Gain1/1 -> Divide/1
  Product7/1 -> Ph/1
  Product6/1 -> Display1/1, rhoh/1

== system WindFoR_model/Subsystem1/Dynamics_EoM/Force_Dynamics_WindAxis/BodyToWind ==
  alpha : Inport
  beta : Inport  Port=2
  Product : Product  Multiplication=Matrix(*)
  Subsystem5 : Subsystem
  Subsystem7 : Subsystem
  Transpose : Math  Operator=transpose
  R_BW : Outport
  wires:
  beta/1 -> Subsystem7/1(beta)
  Product/1 -> Transpose/1
  Subsystem5/1(R_alpha) -> Product/1
  Subsystem7/1(R_beta) -> Product/2
  alpha/1 -> Subsystem5/1(alpha)
  Transpose/1 -> R_BW/1

== system WindFoR_model/Subsystem1/Dynamics_EoM/Force_Dynamics_WindAxis/Subsystem ==
  alpha : Inport
  Constant1 : Constant
  Constant{2..4,6..7} (5 alike) : Constant  Value=0
  Constant5 : Constant
  Gain : Gain  Gain=-1
  Mux2 : Mux  Inputs=9
  Reshape : Reshape  OutputDimensionality=Customize  OutputDimensions=[3,3]
  Sin1 : Trigonometry
  Sin2 : Trigonometry  Operator=cos
  Transpose : Math  Operator=transpose
  R_rate_bw : Outport
  wires:
  Sin2/1 -> Mux2/9
  Gain/1 -> Mux2/7
  Reshape/1 -> Transpose/1
  Sin1/1 -> Gain/1
  Constant1/1 -> Mux2/1
  Constant4/1 -> Mux2/4
  alpha/1 -> Sin2/1, Sin1/1
  Mux2/1 -> Reshape/1
  Constant7/1 -> Mux2/8
  Constant3/1 -> Mux2/3
  Constant5/1 -> Mux2/5
  Constant2/1 -> Mux2/2
  Constant6/1 -> Mux2/6
  Transpose/1 -> R_rate_bw/1  "R_rate_bw"

== system WindFoR_model/Subsystem1/Dynamics_EoM/Force_Dynamics_WindAxis/BodyToWind/Subsystem5 ==
  note: Reshape creates array by arranging them in column first manner
  alpha : Inport
  Constant{,1,3..4} (4 alike) : Constant  Value=0
  Constant2 : Constant
  Cos3 : Trigonometry  Operator=cos
  Gain : Gain  Gain=-1
  Mux : Mux  Inputs=9
  Reshape : Reshape  OutputDimensionality=Customize  OutputDimensions=[3,3]
  Sin3 : Trigonometry
  Transpose : Math  Operator=transpose
  R_alpha : Outport
  wires:
  Transpose/1 -> R_alpha/1
  [sinALPHA] -> Gain/1
  Constant3/1 -> Mux/6
  Constant/1 -> Mux/2
  [cosALPHA] -> Mux/1
  Reshape/1 -> Transpose/1
  Mux/1 -> Reshape/1
  Cos3/1 -> [cosALPHA]
  Sin3/1 -> [sinALPHA]
  [cosALPHA] -> Mux/9
  alpha/1 -> Cos3/1, Sin3/1
  Gain/1 -> Mux/3
  Constant1/1 -> Mux/4
  [sinALPHA] -> Mux/7
  Constant2/1 -> Mux/5
  Constant4/1 -> Mux/8

== system WindFoR_model/Subsystem1/Dynamics_EoM/Force_Dynamics_WindAxis/BodyToWind/Subsystem7 ==
  note: Reshape creates array by arranging them in column first manner
  beta : Inport
  Constant{5..6,8..9} (4 alike) : Constant  Value=0
  Constant7 : Constant
  Cos4 : Trigonometry  Operator=cos
  Gain2 : Gain  Gain=-1
  Mux1 : Mux  Inputs=9
  Reshape1 : Reshape  OutputDimensionality=Customize  OutputDimensions=[3,3]
  Sin4 : Trigonometry
  Transpose : Math  Operator=transpose
  R_beta : Outport
  wires:
  Transpose/1 -> R_beta/1
  [cosBETA] -> Mux1/5
  Constant7/1 -> Mux1/9
  beta/1 -> Cos4/1, Sin4/1
  Cos4/1 -> [cosBETA]
  Constant6/1 -> Mux1/7
  Sin4/1 -> [sinBETA]
  Gain2/1 -> Mux1/4
  Constant8/1 -> Mux1/6
  [cosBETA] -> Mux1/1
  [sinBETA] -> Mux1/2
  Constant5/1 -> Mux1/3
  Constant9/1 -> Mux1/8
  Reshape1/1 -> Transpose/1
  Mux1/1 -> Reshape1/1
  [sinBETA] -> Gain2/1
